simulink library "EV_VLD"  (R2019b)
settings: Solver=VariableStepAuto  StartTime=0.0  StopTime=10.0  RelTol=1e-3
undefined symbols (not defined in the file): DiscIntNeverNeededParam
libraries: $bdroot x2, simulink x2
(part 2 of 2)

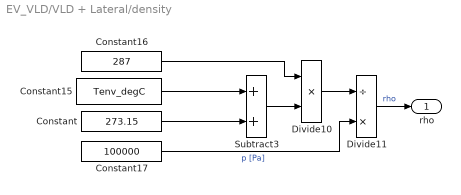
== system EV_VLD/VLD + Lateral/density ==
  Constant : Constant  Value=273.15
  Constant15 : Constant  Value=Tenv_degC
  Constant16 : Constant  Value=287
  Constant17 : Constant  Value=100000
  Divide10 : Product
  Divide11 : Product  Inputs=/*
  Subtract3 : Sum
  rho : Outport
  wires:
  Subtract3/1 -> Divide10/2
  Divide11/1 -> rho/1  "rho"
  Constant16/1 -> Divide10/1
  Constant15/1 -> Subtract3/1
  Constant17/1 -> Divide11/2  "p [Pa]"
  Constant/1 -> Subtract3/2
  Divide10/1 -> Divide11/1

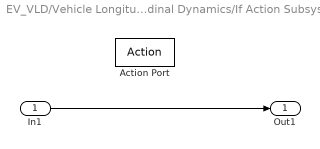
== system EV_VLD/Vehicle Longitudinal Dynamics/If Action Subsystem ==
  In1 : Inport
  Action Port : ActionPort  ActionPortLabel=else
  Out1 : Outport
  wires:
  In1/1 -> Out1/1

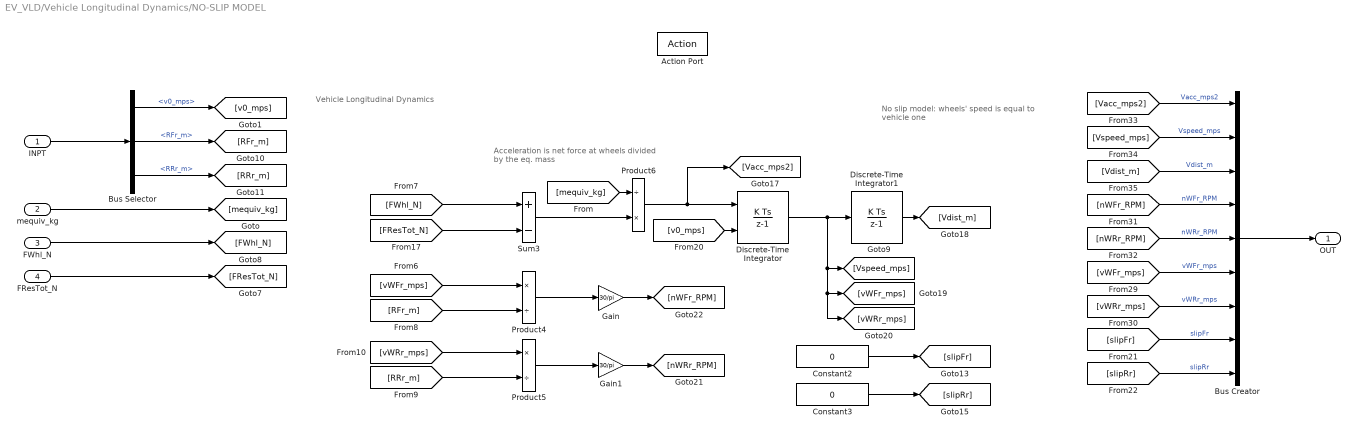
== system EV_VLD/Vehicle Longitudinal Dynamics/NO-SLIP MODEL ==
  note: Vehicle Longitudinal Dynamics
  note: No slip model: wheels' speed is equal to vehicle one
  note: Acceleration is net force at wheels divided by the eq. mass
  INPT : Inport
  mequiv_kg : Inport  Port=2
  FWhl_N : Inport  Port=3
  FResTot_N : Inport  Port=4
  Action Port : ActionPort  ActionPortLabel=if(u1 == 0)
  Bus Creator : BusCreator  Inputs=9
  Bus Selector : BusSelector  OutputSignals=v0_mps,RFr_m,RRr_m
  Constant2 : Constant  Value=0
  Constant3 : Constant  Value=0
  Discrete-Time Integrator : DiscreteIntegrator  InitialConditionSource=external  SampleTime=-1  LimitOutput=on  LowerSaturationLimit=1e-3  ICPrevOutput=DiscIntNeverNeededParam  ICPrevScaledInput=DiscIntNeverNeededParam
  Discrete-Time Integrator1 : DiscreteIntegrator  InitialCondition=1e-6  SampleTime=-1  LowerSaturationLimit=0  ICPrevOutput=DiscIntNeverNeededParam  ICPrevScaledInput=DiscIntNeverNeededParam
  Gain : Gain  Gain=30/pi
  Gain1 : Gain  Gain=30/pi
  Product4 : Product  Inputs=*/
  Product5 : Product  Inputs=*/
  Product6 : Product  Inputs=/*
  Sum3 : Sum  Inputs=+-
  OUT : Outport
  wires:
  [Vspeed_mps] -> Bus Creator/2  "Vspeed_mps"
  [vWFr_mps] -> Bus Creator/6  "vWFr_mps"
  [vWRr_mps] -> Bus Creator/7  "vWRr_mps"
  [Vdist_m] -> Bus Creator/3  "Vdist_m"
  [v0_mps] -> Discrete-Time Integrator/2
  Discrete-Time Integrator/1 -> [vWFr_mps], [vWRr_mps], [Vspeed_mps], Discrete-Time Integrator1/1
  [slipRr] -> Bus Creator/9  "slipRr"
  [FWhl_N] -> Sum3/1
  [nWRr_RPM] -> Bus Creator/5  "nWRr_RPM"
  [mequiv_kg] -> Product6/1
  [FResTot_N] -> Sum3/2
  Bus Selector/3 -> [RRr_m]  "<RRr_m>"
  Bus Selector/1 -> [v0_mps]  "<v0_mps>"
  INPT/1 -> Bus Selector/1
  Bus Selector/2 -> [RFr_m]  "<RFr_m>"
  [Vacc_mps2] -> Bus Creator/1  "Vacc_mps2"
  [nWFr_RPM] -> Bus Creator/4  "nWFr_RPM"
  Bus Creator/1 -> OUT/1
  Discrete-Time Integrator1/1 -> [Vdist_m]
  Gain/1 -> [nWFr_RPM]
  [slipFr] -> Bus Creator/8  "slipFr"
  Gain1/1 -> [nWRr_RPM]
  [vWRr_mps] -> Product5/1
  [RRr_m] -> Product5/2
  [vWFr_mps] -> Product4/1
  [RFr_m] -> Product4/2
  Product4/1 -> Gain/1
  Product5/1 -> Gain1/1
  Constant2/1 -> [slipFr]
  Constant3/1 -> [slipRr]
  mequiv_kg/1 -> [mequiv_kg]
  FWhl_N/1 -> [FWhl_N]
  FResTot_N/1 -> [FResTot_N]
  Product6/1 -> Discrete-Time Integrator/1, [Vacc_mps2]
  Sum3/1 -> Product6/2

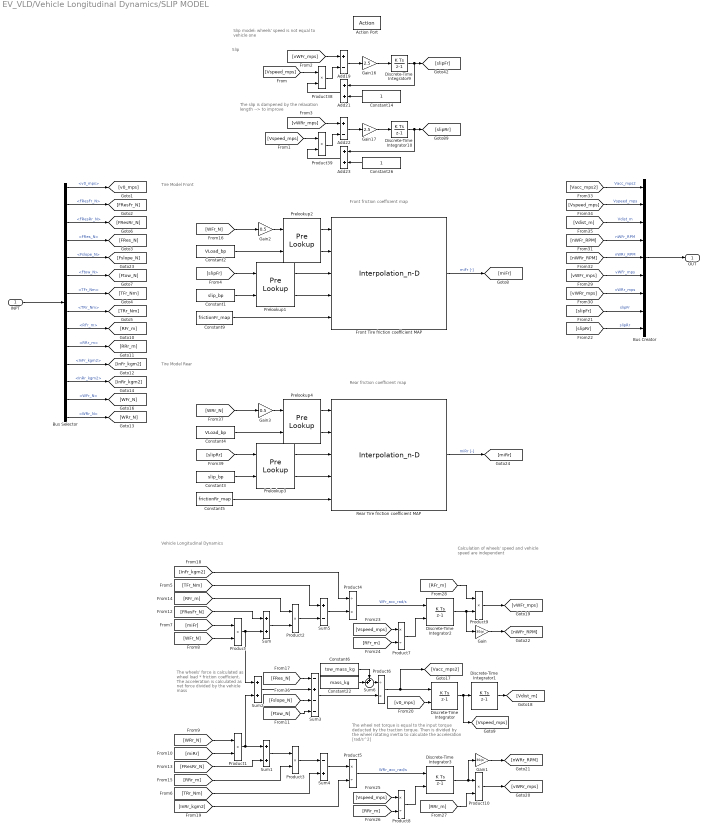
== system EV_VLD/Vehicle Longitudinal Dynamics/SLIP MODEL ==
  note: Tire Model Front
  note: Slip
  note: Vehicle Longitudinal Dynamics
  note: Tire Model Rear
  note: Slip model: wheels' speed is not equal to vehicle one
  note: The slip is dampened by the relaxation length --> to improve
  note: Front friction coefficient map
  note: Rear friction coefficient map
  note: The wheels' force is calculated as wheel load * friction coefficient. The acceleration is calculated as net force divided by the vehicle mass
  note: Calculation of wheels' speed and vehicle speed are independent
  note: The wheel net torque is equal to the input torque deducted by the traction torque. Then is divided by the wheel rotating inertia to calculate the acceleration [rad/s^2]
  INPT : Inport
  Action Port : ActionPort  ActionPortLabel=else
  Add19 : Sum  Inputs=+-
  Add21 : Sum
  Add22 : Sum  Inputs=+-
  Add23 : Sum
  Bus Creator : BusCreator  Inputs=9
  Bus Selector : BusSelector  OutputSignals=v0_mps,FResFr_N,FResRr_N,FRes_N,Fslope_N,Ftow_N,TFr_Nm,TRr_Nm,RFr_m,RRr_m,InFr_kgm2,InRr_kgm2,WFr_N,WRr_N
  Constant1 : Constant  Value=slip_bp
  Constant14 : Constant
  Constant2 : Constant  Value=VLoad_bp
  Constant22 : Constant  Value=mass_kg
  Constant26 : Constant
  Constant3 : Constant  Value=slip_bp
  Constant4 : Constant  Value=VLoad_bp
  Constant5 : Constant  Value=frictionRr_map
  Constant6 : Constant  Value=tow_mass_kg
  Constant9 : Constant  Value=frictionFr_map
  Discrete-Time Integrator : DiscreteIntegrator  InitialConditionSource=external  SampleTime=-1  LimitOutput=on  LowerSaturationLimit=1e-3  ICPrevOutput=DiscIntNeverNeededParam  ICPrevScaledInput=DiscIntNeverNeededParam
  Discrete-Time Integrator1 : DiscreteIntegrator  InitialCondition=1e-6  SampleTime=-1  LowerSaturationLimit=0  ICPrevOutput=DiscIntNeverNeededParam  ICPrevScaledInput=DiscIntNeverNeededParam
  Discrete-Time Integrator10 : DiscreteIntegrator  gainval=1  SampleTime=-1  LimitOutput=on  UpperSaturationLimit=1  LowerSaturationLimit=-1  ICPrevOutput=DiscIntNeverNeededParam  ICPrevScaledInput=DiscIntNeverNeededParam
  Discrete-Time Integrator2 : DiscreteIntegrator  InitialConditionSource=external  SampleTime=-1  LimitOutput=on  LowerSaturationLimit=1e-3  ICPrevOutput=DiscIntNeverNeededParam  ICPrevScaledInput=DiscIntNeverNeededParam
  Discrete-Time Integrator3 : DiscreteIntegrator  InitialConditionSource=external  SampleTime=-1  LimitOutput=on  LowerSaturationLimit=1e-3  ICPrevOutput=DiscIntNeverNeededParam  ICPrevScaledInput=DiscIntNeverNeededParam
  Discrete-Time Integrator9 : DiscreteIntegrator  gainval=1  SampleTime=-1  LimitOutput=on  UpperSaturationLimit=1  LowerSaturationLimit=-1  ICPrevOutput=DiscIntNeverNeededParam  ICPrevScaledInput=DiscIntNeverNeededParam
  Front Tire friction coefficient MAP : Interpolation_n-D  TableSource=Input port
      settings: InputPortMap=u0,u1,u2,u3,p2
  Gain : Gain  Gain=30/pi
  Gain1 : Gain  Gain=30/pi
  Gain16 : Gain  Gain=2.5
  Gain17 : Gain  Gain=2.5
  Gain2 : Gain  Gain=0.5
  Gain3 : Gain  Gain=0.5
  Prelookup1 : PreLookup  BreakpointsDataSource=Input port  BreakpointsData=[1:4]  ExtrapMethod=Linear  FractionDataTypeStr=double
      settings: InputPortMap=u0,p1
  Prelookup2 : PreLookup  BreakpointsDataSource=Input port  BreakpointsData=[1:4]  ExtrapMethod=Linear  FractionDataTypeStr=double
      settings: InputPortMap=u0,p1
  Prelookup3 : PreLookup  BreakpointsDataSource=Input port  BreakpointsData=[1:4]  FractionDataTypeStr=double
      settings: InputPortMap=u0,p1
  Prelookup4 : PreLookup  BreakpointsDataSource=Input port  BreakpointsData=[1:4]  ExtrapMethod=Linear  FractionDataTypeStr=double
      settings: InputPortMap=u0,p1
  Product{,1..3,9..10} (6 alike) : Product
  Product38 : Product  Inputs=**
  Product39 : Product  Inputs=**
  Product4 : Product  Inputs=/*
  Product5 : Product  Inputs=*/
  Product6 : Product  Inputs=/*
  Product7 : Product  Inputs=*/
  Product8 : Product  Inputs=*/
  Rear Tire friction coefficient MAP : Interpolation_n-D  TableSource=Input port
      settings: InputPortMap=u0,u1,u2,u3,p2
  Sum : Sum
  Sum1 : Sum
  Sum2 : Sum
  Sum3 : Sum  Inputs=-+--
  Sum4 : Sum  Inputs=-+
  Sum5 : Sum  Inputs=+-
  Sum6 : Sum  Inputs=++|
  OUT : Outport
  wires:
  INPT/1 -> Bus Selector/1
  Bus Selector/1 -> [v0_mps]  "<v0_mps>"
  Bus Selector/2 -> [FResFr_N]  "<FResFr_N>"
  Bus Selector/3 -> [FResRr_N]  "<FResRr_N>"
  Bus Selector/4 -> [FRes_N]  "<FRes_N>"
  Bus Selector/7 -> [TFr_Nm]  "<TFr_Nm>"
  Bus Selector/8 -> [TRr_Nm]  "<TRr_Nm>"
  Bus Selector/9 -> [RFr_m]  "<RFr_m>"
  Bus Selector/10 -> [RRr_m]  "<RRr_m>"
  Bus Selector/11 -> [InFr_kgm2]  "<InFr_kgm2>"
  Bus Selector/12 -> [InRr_kgm2]  "<InRr_kgm2>"
  Prelookup1/2 -> Front Tire friction coefficient MAP/4
  Prelookup2/1 -> Front Tire friction coefficient MAP/1
  Prelookup2/2 -> Front Tire friction coefficient MAP/2
  [WFr_N] -> Gain2/1
  [slipFr] -> Prelookup1/1
  Front Tire friction coefficient MAP/1 -> [miFr]  "miFr [-]"
  Constant2/1 -> Prelookup2/2
  Prelookup1/1 -> Front Tire friction coefficient MAP/3
  Constant1/1 -> Prelookup1/2
  Bus Selector/13 -> [WFr_N]  "<WFr_N>"
  Bus Selector/14 -> [WRr_N]  "<WRr_N>"
  [miFr] -> Product/1
  [WFr_N] -> Product/2
  [miRr] -> Product1/2
  [WRr_N] -> Product1/1
  Product1/1 -> Sum1/1, Sum2/2
  Product/1 -> Sum/2, Sum2/1
  [FResFr_N] -> Sum/1
  [FResRr_N] -> Sum1/2
  Sum/1 -> Product2/2
  [RFr_m] -> Product2/1
  Sum1/1 -> Product3/1
  [RRr_m] -> Product3/2
  Product3/1 -> Sum4/1
  [TRr_Nm] -> Sum4/2
  Product2/1 -> Sum5/2
  [TFr_Nm] -> Sum5/1
  Sum5/1 -> Product4/2
  Sum4/1 -> Product5/1
  [InFr_kgm2] -> Product4/1
  [InRr_kgm2] -> Product5/2
  Constant22/1 -> Sum6/2
  Sum3/1 -> Product6/2
  Product6/1 -> [Vacc_mps2], Discrete-Time Integrator/1
  [v0_mps] -> Discrete-Time Integrator/2
  Discrete-Time Integrator/1 -> [Vspeed_mps], Discrete-Time Integrator1/1
  Discrete-Time Integrator1/1 -> [Vdist_m]
  Product4/1 -> Discrete-Time Integrator2/1  "WFr_acc_rad/s"
  Product5/1 -> Discrete-Time Integrator3/1  "WRr_acc_rad/s"
  [Vspeed_mps] -> Product7/1
  [RFr_m] -> Product7/2
  [RRr_m] -> Product8/2
  [Vspeed_mps] -> Product8/1
  Product8/1 -> Discrete-Time Integrator3/2
  Product7/1 -> Discrete-Time Integrator2/2
  Discrete-Time Integrator2/1 -> Gain/1, Product9/2
  Discrete-Time Integrator3/1 -> Gain1/1, Product10/1
  [RRr_m] -> Product10/2
  [RFr_m] -> Product9/1
  Product9/1 -> [vWFr_mps]
  Product10/1 -> [vWRr_mps]
  Gain/1 -> [nWFr_RPM]
  Gain1/1 -> [nWRr_RPM]
  [Vacc_mps2] -> Bus Creator/1  "Vacc_mps2"
  [Vspeed_mps] -> Bus Creator/2  "Vspeed_mps"
  [Vdist_m] -> Bus Creator/3  "Vdist_m"
  [nWFr_RPM] -> Bus Creator/4  "nWFr_RPM"
  [nWRr_RPM] -> Bus Creator/5  "nWRr_RPM"
  [vWFr_mps] -> Bus Creator/6  "vWFr_mps"
  [vWRr_mps] -> Bus Creator/7  "vWRr_mps"
  [slipFr] -> Bus Creator/8  "slipFr"
  [slipRr] -> Bus Creator/9  "slipRr"
  Bus Creator/1 -> OUT/1
  Gain2/1 -> Prelookup2/1
  Constant9/1 -> Front Tire friction coefficient MAP/5
  Bus Selector/5 -> [Fslope_N]  "<Fslope_N>"
  Constant5/1 -> Rear Tire friction coefficient MAP/5
  Gain3/1 -> Prelookup4/1
  Constant3/1 -> Prelookup3/2
  Prelookup3/1 -> Rear Tire friction coefficient MAP/3
  Constant4/1 -> Prelookup4/2
  [slipRr] -> Prelookup3/1
  [WRr_N] -> Gain3/1
  Rear Tire friction coefficient MAP/1 -> [miRr]  "miRr [-]"
  Prelookup4/2 -> Rear Tire friction coefficient MAP/2
  Prelookup4/1 -> Rear Tire friction coefficient MAP/1
  Prelookup3/2 -> Rear Tire friction coefficient MAP/4
  [Vspeed_mps] -> Product39/1
  Gain17/1 -> Discrete-Time Integrator10/1
  Gain16/1 -> Discrete-Time Integrator9/1
  Add19/1 -> Gain16/1
  [Vspeed_mps] -> Product38/1
  [vWRr_mps] -> Add22/1
  Add22/1 -> Gain17/1
  Constant26/1 -> Add23/2
  Product39/1 -> Add22/2
  Add23/1 -> Product39/2
  Add21/1 -> Product38/2
  Discrete-Time Integrator10/1 -> Add23/1, [slipRr]
  Product38/1 -> Add19/2
  [vWFr_mps] -> Add19/1
  Constant14/1 -> Add21/2
  Discrete-Time Integrator9/1 -> Add21/1, [slipFr]
  Bus Selector/6 -> [Ftow_N]  "<Ftow_N>"
  [FRes_N] -> Sum3/1
  Sum2/1 -> Sum3/2
  [Fslope_N] -> Sum3/3
  [Ftow_N] -> Sum3/4
  Sum6/1 -> Product6/1
  Constant6/1 -> Sum6/1

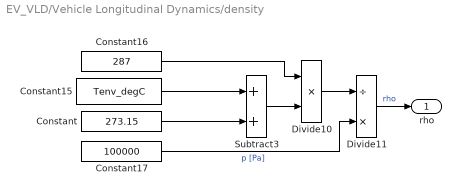
== system EV_VLD/Vehicle Longitudinal Dynamics/density ==
  Constant : Constant  Value=273.15
  Constant15 : Constant  Value=Tenv_degC
  Constant16 : Constant  Value=287
  Constant17 : Constant  Value=100000
  Divide10 : Product
  Divide11 : Product  Inputs=/*
  Subtract3 : Sum
  rho : Outport
  wires:
  Divide10/1 -> Divide11/1
  Constant/1 -> Subtract3/2
  Constant17/1 -> Divide11/2  "p [Pa]"
  Constant15/1 -> Subtract3/1
  Constant16/1 -> Divide10/1
  Divide11/1 -> rho/1  "rho"
  Subtract3/1 -> Divide10/2
